simulink model "m2"  (R2022b)
settings: Solver=VariableStepAuto  StartTime=0.0  StopTime=0.5  RelTol=1e-3
libraries: spsIGBTLib x4, spsSeriesRLCBranchLib x3, spsCurrentMeasurementLib x2, spsDiodeLib x2, spsDCVoltageSourceLib x1, spsLinearTransformerLib x1, spsMeanLib x1, spsVoltageMeasurementLib x1, sps_lib x1
settings Model: Creator=李方超  LastModifiedBy=李方超

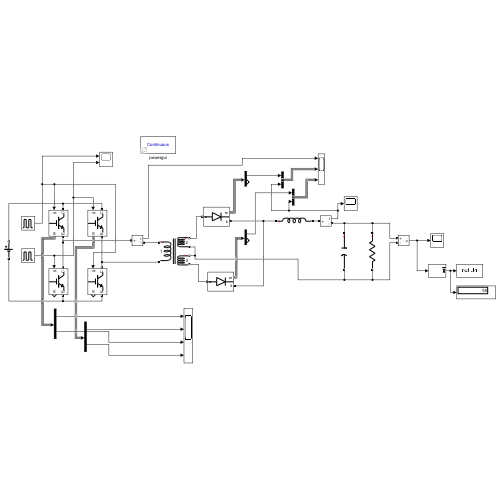
[thumbnail: Simulink's stored preview of the top-level diagram]
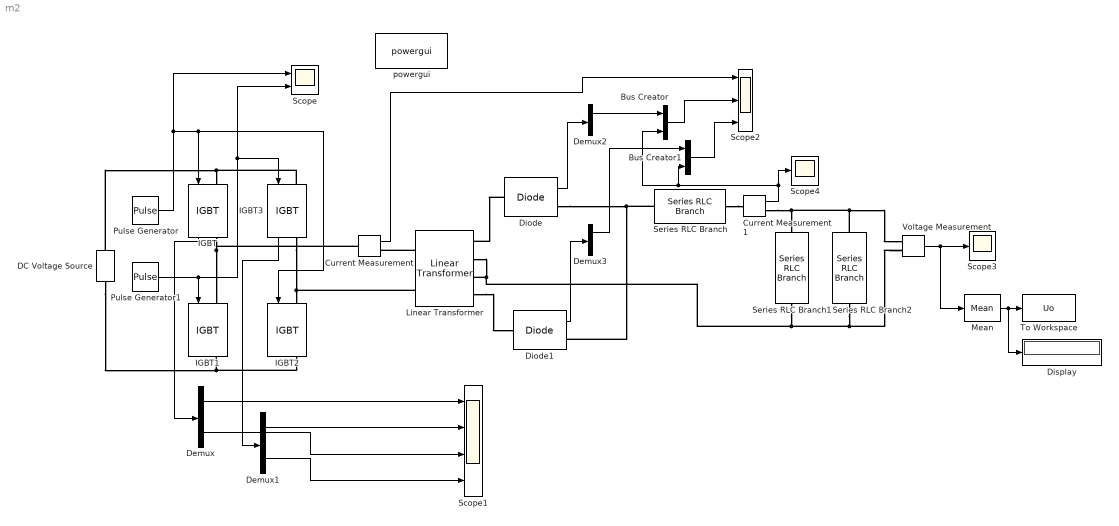
== system m2 ==
  Bus Creator : BusCreator  Inputs=2
  Bus Creator1 : BusCreator  Inputs=2
  Current Measurement : spsCurrentMeasurementLib/Current Measurement  PhasorSimulation=off  OutputType=Complex  PSBequivalent=0
  Current Measurement1 : spsCurrentMeasurementLib/Current Measurement  PhasorSimulation=off  OutputType=Complex  PSBequivalent=0
  DC Voltage Source : spsDCVoltageSourceLib/DC Voltage Source  Amplitude=800  Measurements=None
  Demux{,1..3} (4 alike) : Demux  Outputs=2
  Diode : spsDiodeLib/Diode  Ron=0  Lon=0  Vf=0  IC=0  UseSnubber=0  Rs=inf  Cs=0  Measurements=on
  Diode1 : spsDiodeLib/Diode  Ron=0  Lon=0  Vf=0  IC=0  UseSnubber=0  Rs=inf  Cs=0  Measurements=on
  Display : Display
  IGBT{,1..3} (4 alike) : spsIGBTLib/IGBT  Ron=0  Lon=0  Vf=0  Tf=1e-6  Tt=2e-6  IC=0  Rs=inf  Cs=inf  Measurements=on
  Linear Transformer : spsLinearTransformerLib/Linear Transformer  UNITS=pu  NominalPower=[ 250e6 60 ]  winding1="[ 600e3  0 0 ]"  winding2="[ 100e3  0 0 ]"  ThreeWindings=on  winding3=[ 100e3 0 0 ]  RmLm=[ inf inf ]  Measurements=None  DataType=off
  Mean : spsMeanLib/Mean  Freq=1e5  Vinit=0  Ts=0
  Pulse Generator : DiscretePulseGenerator  PulseType=Time based  Period=1e-5  PulseWidth=300/16
  Pulse Generator1 : DiscretePulseGenerator  PulseType=Time based  Period=1e-5  PulseWidth=300/16  PhaseDelay=5e-6
  Scope : Scope  NumInputPorts=2
  Scope1 : Scope  NumInputPorts=4
  Scope2 : Scope  NumInputPorts=3
  Scope3 : Scope
  Scope4 : Scope
  Series RLC Branch : spsSeriesRLCBranchLib/Series RLC Branch  LConnTagsString=__new0  RConnTagsString=__new0  BranchType=L  Resistance=1  Inductance=600e-6  SetiL0=off  InitialCurrent=0  Capacitance=1e-6  Setx0=off  InitialVoltage=0  Measurements=None
  Series RLC Branch1 : spsSeriesRLCBranchLib/Series RLC Branch  LConnTagsString=__new0  RConnTagsString=__new0  BranchType=C  Resistance=1  Inductance=1e-3  SetiL0=off  InitialCurrent=0  Capacitance=200e-6  Setx0=off  InitialVoltage=0  Measurements=None
  Series RLC Branch2 : spsSeriesRLCBranchLib/Series RLC Branch  LConnTagsString=__new0  RConnTagsString=__new0  BranchType=R  Resistance=60  Inductance=1e-3  SetiL0=off  InitialCurrent=0  Capacitance=200e-6  Setx0=off  InitialVoltage=0  Measurements=None
  To Workspace : ToWorkspace  VariableName=Uo  SaveFormat=Timeseries  SampleTime=-1
  Voltage Measurement : spsVoltageMeasurementLib/Voltage Measurement  PhasorSimulation=off  OutputType=Complex  PSBequivalent=0
  powergui : sps_lib/powergui  Priority=1  SimulationMode=Continuous  SampleTime=1e-7  frequency=60  Iterations=50  frequencyindice=0  Pbase=100e6  ErrMax=1e-4  UnitsV=kV  UnitsW=MW  buscounter=0  FunctionMessages=off  echomessages=off  EnableUseOfTLC=off  CurrentSourceSwitches=off  DisableSnubberDevices=off  DisableRonSwitches=off  DisableVfSwitches=off  DisplayEquations=off  AutomaticDiscreteSolvers=off  SolverType=Tustin/Backward Euler (TBE)  Interpol=off  ExternalGateDelay=off  methode=off  Ts=100  x0status=blocks  SPID=on  SwTol=0  HookPort=off  NonlinearTolerance=1e-4  nMaxIteration=100  ContinueOnMaxIteration=off  RestoreLinks=warning  ResistiveCurrentMeasurement=off  Frange=[0:2:500]  Ylog=off  Xlog=on  ShowGrid=off  save=off  variable=ZData  structure=0  ZoomFFT=off  StartTime=0.0  cycles=1  DisplayStyle=1  fundamental=60  FreqAxis=off  MaxFrequency=1000  frequencyindicesteady=1  RmsSteady=1  display=off
  wires:
  Pulse Generator/1 -> Scope/1, IGBT/1, IGBT2/1
  Pulse Generator1/1 -> IGBT1/1, IGBT3/1, Scope/2
  IGBT/1 -> Demux/1
  Demux/1 -> Scope1/1
  IGBT3/1 -> Demux1/1
  Demux1/1 -> Scope1/2
  Demux/2 -> Scope1/3
  Demux1/2 -> Scope1/4
  Diode/1 -> Demux2/1
  Diode1/1 -> Demux3/1
  Demux2/1 -> Bus Creator/1
  Voltage Measurement/1 -> Mean/1, Scope3/1
  Current Measurement/1 -> Scope2/1
  Current Measurement1/1 -> Bus Creator1/2, Bus Creator/2, Scope4/1
  Bus Creator/1 -> Scope2/2
  Demux3/1 -> Bus Creator1/1
  Bus Creator1/1 -> Scope2/3
  Mean/1 -> Display/1, To Workspace/1
  connections:
  DC Voltage Source/RConn1 -- IGBT3/LConn1 -- IGBT/LConn1
  IGBT/RConn1 -- Current Measurement/LConn1 -- IGBT1/LConn1
  DC Voltage Source/LConn1 -- IGBT2/RConn1 -- IGBT1/RConn1
  IGBT3/RConn1 -- Linear Transformer/LConn2 -- IGBT2/LConn1
  Diode/LConn1 -- Linear Transformer/RConn1
  Linear Transformer/RConn2 -- Series RLC Branch2/RConn1 -- Voltage Measurement/LConn2 -- Series RLC Branch1/RConn1 -- Linear Transformer/RConn3
  Linear Transformer/RConn4 -- Diode1/LConn1
  Diode/RConn1 -- Series RLC Branch/LConn1 -- Diode1/RConn1
  Linear Transformer/LConn1 -- Current Measurement/RConn1
  Series RLC Branch/RConn1 -- Current Measurement1/LConn1
  Series RLC Branch2/LConn1 -- Series RLC Branch1/LConn1 -- Current Measurement1/RConn1 -- Voltage Measurement/LConn1
